simulink model "task_1"  (R2024a)
settings: Solver=FixedStepAuto  StartTime=0.0  StopTime=1  RelTol=1e-3
undefined symbols (not defined in the file): a0, a1, idy, iy
settings Model: Creator=kit  LastModifiedBy=kit

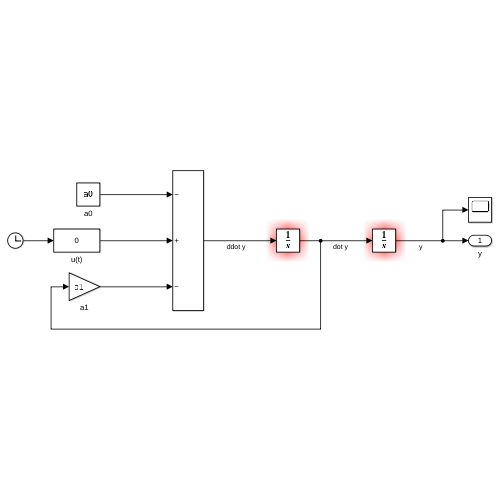
[thumbnail: Simulink's stored preview of the top-level diagram]
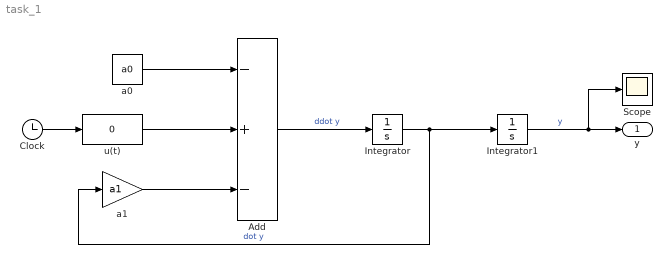
== system task_1 ==
  Add : Sum  Inputs=-+-
  Clock : Clock
  Integrator : Integrator  InitialCondition=idy
  Integrator1 : Integrator  InitialCondition=iy
  Scope : Scope
  a0 : Constant  Value=a0
  a1 : Gain  Gain=a1
  u(t) : Fcn  Expr=0
  y : Outport
  wires:
  Clock/1 -> u(t)/1
  u(t)/1 -> Add/2
  a0/1 -> Add/1
  a1/1 -> Add/3
  Integrator/1 -> a1/1, Integrator1/1  "dot y"
  Add/1 -> Integrator/1  "ddot y"
  Integrator1/1 -> Scope/1, y/1  "y"
